simulink model "FOC_PMSM_FVSensorNew"  (R2019b)
settings: Solver=ode45  StartTime=0  StopTime=1  FixedStep=1/fs/4  MaxStep=1/fs/2  RelTol=1e-7  EnableMultiTasking=on
InitFcn:
  | Motor_parameters_Lsrpm7fw
values from neighbouring files (symbols this model uses):
  c2 = -L2/(L1^2-L2^2)    (= 10.9375)    [Motor_parameters_Lsrpm7fw.m]
  fs = 20e3    (= 20000)    [Motor_parameters_Lsrpm7fw.m]
  Iphmax = I_rated*sqrt(2)*3    [Motor_parameters_Lsrpm7fw.m]
  J = 1*1e-3    (= 0.001)    [Motor_parameters_Lsrpm7fw.m]
  Ki1 = 2    [Motor_parameters_Lsrpm7fw.m]
  Ki2 = 3000    [Motor_parameters_Lsrpm7fw.m]
  Ki_pll = Bw^2*(1.1-0.334*zeta)^2*1/(2*k1)    (= 1705731.55439)    [Motor_parameters_Lsrpm7fw.m]
  Kp1 = 0.005    [Motor_parameters_Lsrpm7fw.m]
  Kp2 = 2    [Motor_parameters_Lsrpm7fw.m]
  Kp_pll = Bw*(2.2*zeta-0.668*zeta^2)*1/(2*k1)    (= 27920.01984)    [Motor_parameters_Lsrpm7fw.m]
  Ld = 10e-3    (= 0.01)    [Motor_parameters_Lsrpm7fw.m]
  Lndd_ini = Lndmpm    (= 0.412)    [Motor_parameters_Lsrpm7fw.m]
  Lndmpm = 0.412    [Motor_parameters_Lsrpm7fw.m]
  Lq = 12.8e-3    (= 0.0128)    [Motor_parameters_Lsrpm7fw.m]
  Npp = 8/2    (= 4)    [Motor_parameters_Lsrpm7fw.m]
  Omegae_ini = 0    [Motor_parameters_Lsrpm7fw.m]
  Rs = 0.78    [Motor_parameters_Lsrpm7fw.m]
  Tl_const = Trat/nrat^2    (= 3.26530612245e-06)    [Motor_parameters_Lsrpm7fw.m]
  Trat = 10    [Motor_parameters_Lsrpm7fw.m]
  Vm = 70    [Motor_parameters_Lsrpm7fw.m]
  Vph = Vs*sqrt(2)    [Motor_parameters_Lsrpm7fw.m]
  wo = 15    [Motor_parameters_Lsrpm7fw.m]
undefined symbols (not defined in the file or in its folder): DiscIntNeverNeededParam, plecs, sigbuilder_block
libraries: simulink x1
(part 1 of 2)
settings Model: Creator=klu  LastModifiedBy=Kristina
settings SolverCC: AlgebraicLoopSolver=LineSearch
settings DataIOCC: LimitDataPoints=on  SaveFormat=Array  SignalLoggingSaveFormat=ModelDataLogs  ReturnWorkspaceOutputs=off
settings OptimizationCC: BooleanDataType=off  ExpressionDepthLimit=2147483647  InitFltsAndDblsToZero=on  LifeSpan=inf
settings DebuggingCC: AlgebraicLoopMsg=none  SaveWithParameterizedLinksMsg=none  UnderspecifiedInitializationDetection=Classic  MergeDetectMultiDrivingBlocksExec=none  SignalResolutionControl=TryResolveAllWithWarning  MultiTaskDSMMsg=warning  MultiTaskCondExecSysMsg=none  FcnCallInpInsideContextMsg=warning  StateNameClashWarn=warning  SFUnexpectedBacktrackingDiag=warning  SFNoUnconditionalDefaultTransitionDiag=warning  SFExecutionAtInitializationDiag=none  ArithmeticOperatorsInVariantConditions=warning
settings HardwareCC: ProdBitPerPointer=32  ProdBitPerSizeT=32  ProdBitPerPtrDiffT=32  ProdLargestAtomicFloat=None  ProdIntDivRoundTo=Undefined  ProdEndianess=Unspecified  ProdWordSize=32  ProdHWDeviceType=32-bit Generic
settings ModelReferenceCC: PropagateSignalLabelsOutOfModel=off
settings SFSimCC: SimUseLocalCustomCode=off  CustomCodeUndefinedFunction=UseInterfaceOnly
settings RTWCC: RTWUseLocalCustomCode=off
settings CodeAppCC: StateflowObjectComments=on
settings GRTTargetCC: TargetFcnLib=ansi_tfl_tmw.mat  TargetLangStandard=C89/C90 (ANSI)  GeneratePreprocessorConditionals=Disable all  CombineOutputUpdateFcns=off  GRTInterface=on
settings ConfigComp: CovMetricSettings=dw  CovHtmlReporting=on  CovSaveCumulativeToWorkspaceVar=on  CovSaveSingleToWorkspaceVar=on  CovExternalEMLEnable=off  CovSFcnEnable=off

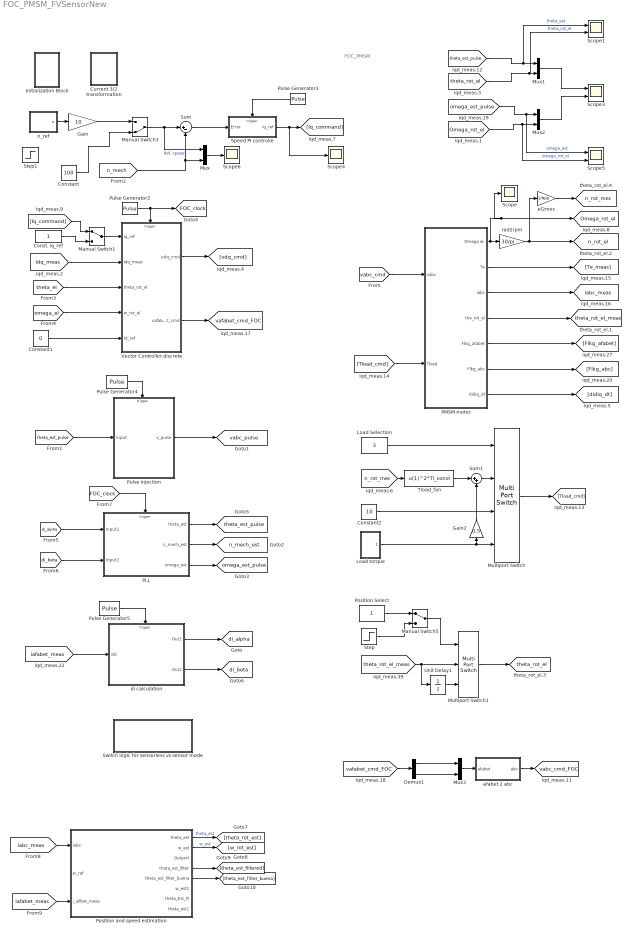
== system FOC_PMSM_FVSensorNew ==
  note: FOC_PMSM
  Const. iq_ref : Constant
  Constant : Constant  Value=100
  Constant1 : Constant  Value=0
  Constant2 : Constant  Value=10
  Current 3/2 transformation : Subsystem
      mask Display:
      | plot([0.1000    0.1357    0.1714    0.2071    0.2429    0.2786    0.3143    0.3500    0.3857    0.4214 0.4571    0.4929    0.5286    0.5643    0.6000]-0.05,0.4+0.6*[0.5000    0.5868    0.6564    0.6950    0.6950    0.6564    0.5868    0.5000    0.4132    0.3436 0.3050    0.3050    0.3436    0.4132    0.5000])
      | 
      | plot([0.1,0.9],[0.1,0.9])
      | 
      | plot([0.5,0.9],0.3*[1 1])
  Demux1 : Demux  Outputs=2
  Gain : Gain  Gain=10
  Gain2 : Gain  Gain=0.5
  Initialization Block : Subsystem  mask{init_in=Motor_parameters_Lsrpm7fw}
      mask prompts: init_in "Enter Initialization Script:"
      mask init:
      | aaa =3;
      mask Callback init_in:
      | init_script=get_param(gcb,'MaskValueString');
      | %eval(init_script);
      | %set_param(gcs,'PreLoadFcn',init_script)
      | set_param(gcs,'InitFcn',init_script)
      | 
      | % Change the parameters here;
      | Ld               = Ld;
      | Lq               = Ld;
  Load Selection : Constant  Value=3
  Load torque : Subsystem
  Manual Switch1 : ManualSwitch
  Manual Switch3 : ManualSwitch  CurrentSetting=0
  Manual Switch5 : ManualSwitch
  Multiport Switch : MultiPortSwitch
  Multiport Switch1 : MultiPortSwitch  Inputs=2
  Mux{,1..3} (4 alike) : Mux  Inputs=2
  PLL : Subsystem  TreatAsAtomicUnit=on
  PMSM motor : Subsystem
  Position Select : Constant
  Position and speed estimation : Subsystem  TreatAsAtomicUnit=on
  Pulse Generator2 : DiscretePulseGenerator  PulseType=Time based  Period=1/fs  PulseWidth=50
  Pulse Generator3 : DiscretePulseGenerator  PulseType=Time based  Period=1/fs  PulseWidth=50
  Pulse Generator4 : DiscretePulseGenerator  PulseType=Time based  Period=1/fs  PulseWidth=50  PhaseDelay=(1/fs)*0.5
  Pulse Generator5 : DiscretePulseGenerator  PulseType=Time based  Period=1/(fs*2)  PulseWidth=50
  Pulse injection : Subsystem  TreatAsAtomicUnit=on
  Scope : Scope
  Scope1 : Scope  NumInputPorts=2
  Scope3 : Scope  NumInputPorts=2
  Scope4 : Scope
  Scope5 : Scope  NumInputPorts=2
  Scope6 : Scope
  Speed PI controlle : Subsystem
  Step : Step  Time=0  Before=1  After=2  SampleTime=0
  Step1 : Step  Time=0.2  Before=100  After=100  SampleTime=0
  Sum : Sum  Inputs=|+-
  Sum1 : Sum  Inputs=|++
  Switch logic for sensorless vs sensor mode : Subsystem
  Tload_fan : Fcn  Expr=u(1)^2*Tl_const
  Unit Delay1 : UnitDelay  SampleTime=(1/fs)*4  HasFrameUpgradeWarning=on
  Vector Controller.discrete : Subsystem
  afabet 2 abc : Subsystem
  di calculation : Subsystem  TreatAsAtomicUnit=on
  el2mec : Gain  Gain=1/Npp
  n_ref : Subsystem  Tag=STV Subsys  LoadFcn=sigbuilder_block('load');  StartFcn=sigbuilder_block('start');  StopFcn=sigbuilder_block('stop');  ClipboardFcn=sigbuilder_block('clipboard');  mask(Sigbuilder block){tuvar=[0:10]}
      mask help: Sigbuilder GUI
      mask init:
      | if ~strcmp(get_param(bdroot(gcbh),'SimulationStatus'),'stopped') tuvar = sigbuilder_block('maskInit'); end
      settings: CopyFcn=sigbuilder_block('copy');  DeleteFcn=sigbuilder_block('delete');  ModelCloseFcn=sigbuilder_block('modelClose');  PreSaveFcn=sigbuilder_block('preSave');  PauseFcn=sigbuilder_block('pause')  ContinueFcn=sigbuilder_block('continue')  NameChangeFcn=sigbuilder_block('namechange');  OpenFcn=sigbuilder_block('open',[72.75 116.25 550.5 363.75 ]);  CloseFcn=sigbuilder_block('close');
      mask Display: plot(0, 0, 100, 100,[2, 2, 32, 32, 2], [68, 8, 8, 68, 68],[32, 2], [38, 38], [32, 19, 2],[53, 60, 44], [32, 17, 17, 2],[16, 16, 31, 31]);txt = getActiveGroup(gcbh);text(2, 100, txt,'verticalAlignment', 'top');
  rad2rpm : Gain  Gain=30/pi
  tag scope: FOC_clock=global, Omega_rot_el=global, di_alpha=global, di_beta=global, iabc_meas=global, n_mech_est=global, n_rot_el=global, n_rot_mec=global, omega_est_pulse=global, theta_est_pulse=global, theta_rot_el=global, theta_rot_el_meas=global, vabc_cmd_FOC=global, vabc_pulse=global, vafabet_cmd_FOC=global
  wires:
  Manual Switch1/1 -> Vector Controller.discrete/1(iq_ref)
  Const. iq_ref/1 -> Manual Switch1/2
  Sum/1 -> Speed PI controlle/1(Error)
  [idq_meas] -> Vector Controller.discrete/2(idq_meas)
  Vector Controller.discrete/1(udq_cmd) -> [vdq_cmd]
  Vector Controller.discrete/2(uafabet_cmd) -> [vafabet_cmd_FOC]
  Constant2/1 -> Multiport Switch/3
  Load torque/1(T_load) -> Multiport Switch/4, Gain2/1
  Multiport Switch/1 -> [Tload_cmd]
  [n_rot_mec] -> Tload_fan/1
  Load Selection/1 -> Multiport Switch/1
  [theta_rot_el_meas] -> Unit Delay1/1, Multiport Switch1/2
  Multiport Switch1/1 -> [theta_rot_el]
  Position Select/1 -> Manual Switch5/1
  Step/1 -> Manual Switch5/2
  Manual Switch5/1 -> Multiport Switch1/1
  n_ref/1(n) -> Gain/1
  Gain/1 -> Manual Switch3/1
  Sum1/1 -> Multiport Switch/2
  Tload_fan/1 -> Sum1/1
  [theta_el] -> Vector Controller.discrete/3(theta_rot_el)
  Constant1/1 -> Vector Controller.discrete/5(Id_ref)
  Gain2/1 -> Sum1/2
  Unit Delay1/1 -> Multiport Switch1/3
  [omega_el] -> Vector Controller.discrete/4(w_rot_el)
  PMSM motor/2(Te) -> [Te_meas]
  PMSM motor/1(Omega el.) -> Scope/1, [Omega_rot_el], rad2rpm/1
  rad2rpm/1 -> [n_rot_el], el2mec/1
  PMSM motor/5(Flkg_afabet) -> [Flkg_afabet]
  PMSM motor/6(Flkg_abc) -> [Flkg_abc]
  [Tload_cmd] -> PMSM motor/2(Tload)
  PMSM motor/3(iabc) -> [iabc_meas]
  PMSM motor/7(didiq_dt) -> [didiq_dt]
  Demux1/2 -> Mux3/2
  Demux1/1 -> Mux3/1
  [vafabet_cmd_FOC] -> Demux1/1
  afabet 2 abc/1(abc) -> [vabc_cmd_FOC]
  Mux3/1 -> afabet 2 abc/1(afabet)
  Speed PI controlle/1(iq_ref) -> Scope4/1, [Iq_command]
  [Iq_command] -> Manual Switch1/1
  el2mec/1 -> [n_rot_mec]
  Pulse Generator3/1 -> Speed PI controlle/Trigger
  Pulse Generator4/1 -> Pulse injection/Trigger
  Pulse Generator2/1 -> [FOC_clock], Vector Controller.discrete/Trigger
  [iafabet_meas] -> di calculation/1(iab)
  Pulse injection/1(v_pulse) -> [vabc_pulse]
  Manual Switch3/1 -> Mux/1, Sum/1  "Ref. speed"
  Mux/1 -> Scope6/1
  [n_mech] -> Mux/2, Sum/2
  [vabc_cmd] -> PMSM motor/1(vabc)
  Pulse Generator5/1 -> di calculation/Trigger
  PMSM motor/4(the_rot_el) -> [theta_rot_el_meas]
  PLL/1(theta_est) -> [theta_est_pulse]
  PLL/2(n_mech_est) -> [n_mech_est]
  PLL/3(omega_est) -> [omega_est_pulse]
  [theta_est_pulse] -> Pulse injection/1(Input)
  di calculation/1(Out1) -> [di_alpha]
  di calculation/2(Out2) -> [di_beta]
  [di_alpha] -> PLL/1(Input1)
  [di_beta] -> PLL/2(Input2)
  [FOC_clock] -> PLL/Trigger
  [theta_est_pulse] -> Scope1/1, Mux1/1  "theta_est"
  [theta_rot_el] -> Scope1/2, Mux1/2  "theta_rot_el"
  [omega_est_pulse] -> Scope5/1, Mux2/1  "omega_est"
  [Omega_rot_el] -> Scope5/2, Mux2/2  "omega_rot_el"
  Mux1/1 -> Scope3/1
  Mux2/1 -> Scope3/2
  Constant/1 -> Manual Switch3/2
  Position and speed estimation/2(w_est) -> [w_rot_est]  "w_est"
  Position and speed estimation/1(theta_est) -> [theta_rot_est]  "theta_est"
  Position and speed estimation/4(theta_est_filter) -> [theta_est_filtered]
  [iabc_meas] -> Position and speed estimation/1(Iabc)
  Position and speed estimation/5(theta_est_filter_buena) -> [theta_est_filter_buena]
  [iafabet_meas] -> Position and speed estimation/3(i_alfbet_meas)

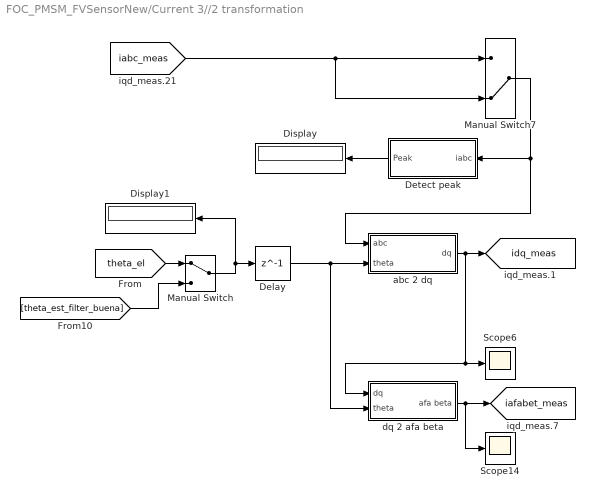
== system FOC_PMSM_FVSensorNew/Current 3//2 transformation ==
  Delay : Delay  DelayLength=1
  Detect peak : Subsystem
  Display : Display
  Display1 : Display
  Manual Switch : ManualSwitch
  Manual Switch7 : ManualSwitch  CurrentSetting=0
  Scope14 : Scope
  Scope6 : Scope
  abc 2 dq : Subsystem
  dq 2 afa beta : Subsystem
  tag scope: iafabet_meas=global, idq_meas=global
  wires:
  abc 2 dq/1(dq) -> [idq_meas], Scope6/1, dq 2 afa beta/1(dq)
  dq 2 afa beta/1(afa beta) -> [iafabet_meas], Scope14/1
  Manual Switch7/1 -> abc 2 dq/1(abc), Detect peak/1(iabc)
  Detect peak/1(Peak) -> Display/1
  [iabc_meas] -> Manual Switch7/1, Manual Switch7/2
  Delay/1 -> abc 2 dq/2(theta), dq 2 afa beta/2(theta)
  [theta_el] -> Manual Switch/1
  Manual Switch/1 -> Display1/1, Delay/1
  [theta_est_filter_buena] -> Manual Switch/2

== system FOC_PMSM_FVSensorNew/Initialization Block ==

== system FOC_PMSM_FVSensorNew/Load torque ==
  Add : Sum  Inputs=+++
  Scope2 : Scope
  Step Load torque 1 : Step  Time=2  After=Trat  SampleTime=0
  Step Load torque2 : Step  Time=4  After=-Trat/2  SampleTime=0
  Tload : Constant  Value=0
  T_load : Outport  VectorParamsAs1DForOutWhenUnconnected=off
  wires:
  Tload/1 -> Add/1
  Step Load torque 1/1 -> Add/2
  Step Load torque2/1 -> Add/3
  Add/1 -> T_load/1, Scope2/1

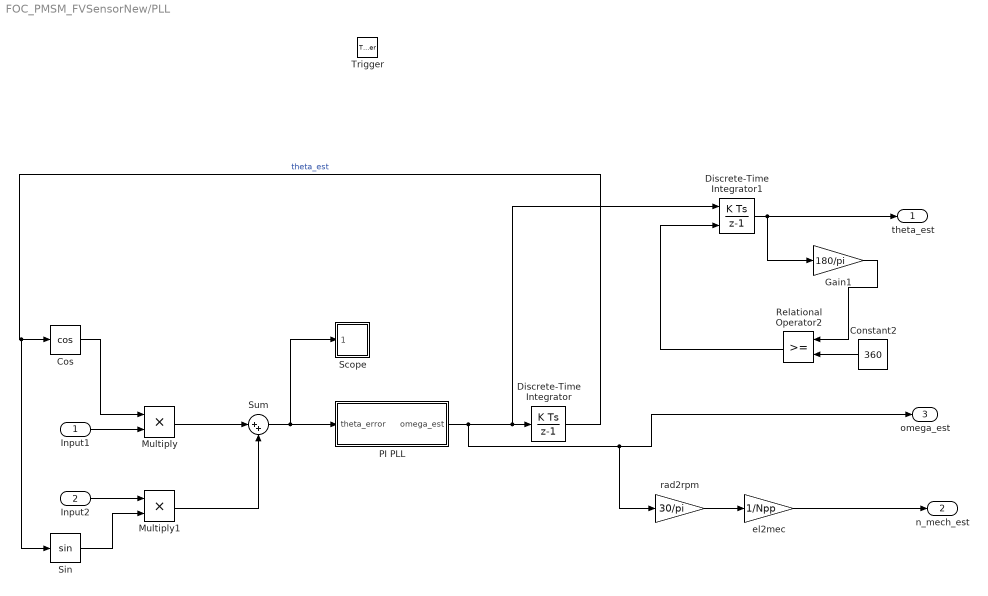
== system FOC_PMSM_FVSensorNew/PLL ==
  Input1 : Inport
  Input2 : Inport  Port=2
  Trigger : TriggerPort  VariantControl=Variant
  Constant2 : Constant  Value=360
  Cos : Trigonometry  Operator=cos
  Discrete-Time Integrator : DiscreteIntegrator  SampleTime=-1  ICPrevOutput=DiscIntNeverNeededParam  ICPrevScaledInput=DiscIntNeverNeededParam
  Discrete-Time Integrator1 : DiscreteIntegrator  ExternalReset=rising  SampleTime=-1  ICPrevOutput=DiscIntNeverNeededParam  ICPrevScaledInput=DiscIntNeverNeededParam
  Gain1 : Gain  Gain=180/pi
  Multiply : Product
  Multiply1 : Product
  PI PLL : Subsystem
  Relational Operator2 : RelationalOperator  OutDataTypeStr=boolean  RndMeth=Nearest
  Scope : Subsystem  LoadFcn=plecs('sl', 300);  InitFcn=plecs('sl', 314);  StartFcn=plecs('sl', 308);  StopFcn=plecs('sl', 309);  mask{Settings=<binary blob, 232 chars, not shown>}
      mask init:
      | plecs('sl', 315);
      settings: CopyFcn=plecs('sl', 303);  DeleteFcn=plecs('sl', 305);  UndoDeleteFcn=plecs('sl', 306);  PreSaveFcn=plecs('sl', 311);  NameChangeFcn=plecs('sl', 310);  DestroyFcn=plecs('sl', 307);  OpenFcn=plecs('sl', 302);  ErrorFcn=plerrorfcn
      mask Display: plot([0.1 0.9 0.9 0.1 0.1], [0.9 0.9 0.5 0.5 0.9])
  Sin : Trigonometry
  Sum : Sum  Inputs=|++
  el2mec : Gain  Gain=1/Npp
  rad2rpm : Gain  Gain=30/pi
  theta_est : Outport  VectorParamsAs1DForOutWhenUnconnected=off
  n_mech_est : Outport  Port=2  VectorParamsAs1DForOutWhenUnconnected=off
  omega_est : Outport  Port=3  VectorParamsAs1DForOutWhenUnconnected=off
  wires:
  el2mec/1 -> n_mech_est/1
  Sum/1 -> Scope/1(1), PI PLL/1(theta_error)
  Multiply/1 -> Sum/1
  Relational Operator2/1 -> Discrete-Time Integrator1/2
  Input2/1 -> Multiply1/1
  Gain1/1 -> Relational Operator2/1
  Discrete-Time Integrator1/1 -> Gain1/1, theta_est/1
  Cos/1 -> Multiply/1
  Sin/1 -> Multiply1/2
  Input1/1 -> Multiply/2
  rad2rpm/1 -> el2mec/1
  Discrete-Time Integrator/1 -> Sin/1, Cos/1  "theta_est"
  PI PLL/1(omega_est) -> rad2rpm/1, omega_est/1, Discrete-Time Integrator1/1, Discrete-Time Integrator/1
  Constant2/1 -> Relational Operator2/2
  Multiply1/1 -> Sum/2

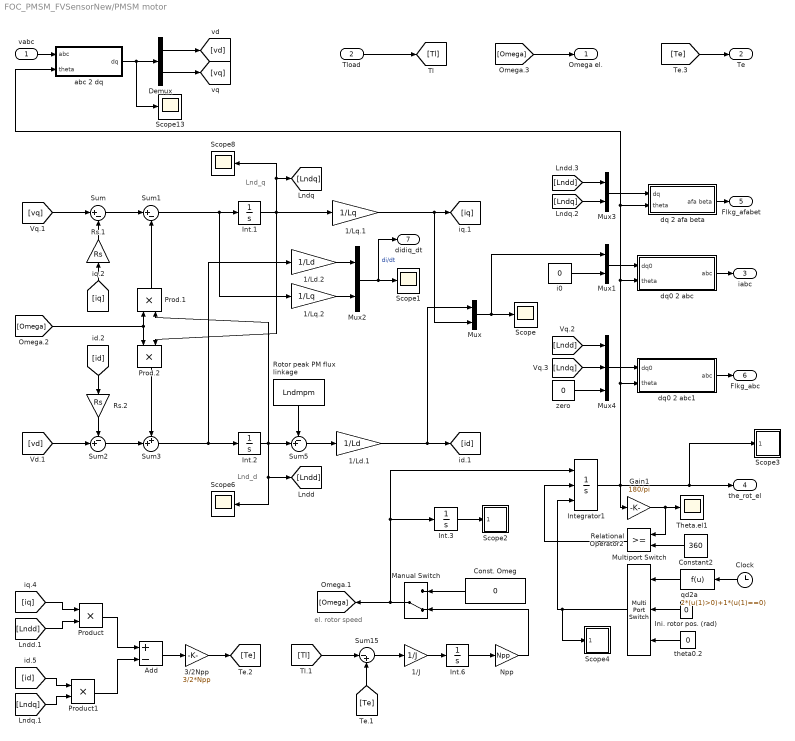
== system FOC_PMSM_FVSensorNew/PMSM motor ==
  note: Lnd_d
  note: Lnd_q
  note: el. rotor speed
  vabc : Inport
  Tload : Inport  Port=2
  1/J : Gain  Gain=1/J
  1/Ld.1 : Gain  Gain=1/Ld
  1/Ld.2 : Gain  Gain=1/Ld
  1/Lq.1 : Gain  Gain=1/Lq
  1/Lq.2 : Gain  Gain=1/Lq
  3/2Npp : Gain  Gain=3/2*Npp
  Add : Sum  Inputs=+-
  Clock : Clock
  Const. Omeg : Constant  Value=0
  Constant2 : Constant  Value=360
  Demux : Demux  Outputs=2
  Gain1 : Gain  Gain=180/pi
  Ini. rotor pos. (rad) : Constant  Value=0
  Int.1 : Integrator
  Int.2 : Integrator  InitialCondition=Lndd_ini
  Int.3 : Integrator  InitialCondition=Omegae_ini/Npp
  Int.6 : Integrator  InitialCondition=Omegae_ini/Npp
  Integrator1 : Integrator  ExternalReset=rising  InitialConditionSource=external  InitialCondition=pi/3
  Manual Switch : ManualSwitch  CurrentSetting=0
  Multiport Switch : MultiPortSwitch  Inputs=2
  Mux{,1..3} (4 alike) : Mux  Inputs=2
  Mux4 : Mux  Inputs=3
  Npp : Gain  Gain=Npp
  Prod.1 : Product  RndMeth=Zero
  Prod.2 : Product  RndMeth=Zero
  Product : Product  RndMeth=Zero
  Product1 : Product  RndMeth=Zero
  Relational Operator2 : RelationalOperator  OutDataTypeStr=boolean  RndMeth=Nearest
  Rotor peak PM flux linkage : Constant  Value=Lndmpm
  Rs.1 : Gain  Gain=Rs
  Rs.2 : Gain  Gain=Rs
  Scope{,1,6,8,13} (5 alike) : Scope
  Scope2 : Subsystem  LoadFcn=plecs('sl', 300);  InitFcn=plecs('sl', 314);  StartFcn=plecs('sl', 308);  StopFcn=plecs('sl', 309);  mask{Settings=<binary blob, 1052 chars, not shown>}
      mask init:
      | plecs('sl', 315);
      settings: CopyFcn=plecs('sl', 303);  DeleteFcn=plecs('sl', 305);  UndoDeleteFcn=plecs('sl', 306);  PreSaveFcn=plecs('sl', 311);  NameChangeFcn=plecs('sl', 310);  DestroyFcn=plecs('sl', 307);  OpenFcn=plecs('sl', 302);  ErrorFcn=plerrorfcn
      mask Display: plot([0.1 0.9 0.9 0.1 0.1], [0.9 0.9 0.5 0.5 0.9])
  Scope3 : Subsystem  LoadFcn=plecs('sl', 300);  InitFcn=plecs('sl', 314);  StartFcn=plecs('sl', 308);  StopFcn=plecs('sl', 309);  mask{Settings=<binary blob, 1052 chars, not shown>}
      mask init:
      | plecs('sl', 315);
      settings: CopyFcn=plecs('sl', 303);  DeleteFcn=plecs('sl', 305);  UndoDeleteFcn=plecs('sl', 306);  PreSaveFcn=plecs('sl', 311);  NameChangeFcn=plecs('sl', 310);  DestroyFcn=plecs('sl', 307);  OpenFcn=plecs('sl', 302);  ErrorFcn=plerrorfcn
      mask Display: plot([0.1 0.9 0.9 0.1 0.1], [0.9 0.9 0.5 0.5 0.9])
  Scope4 : Subsystem  LoadFcn=plecs('sl', 300);  InitFcn=plecs('sl', 314);  StartFcn=plecs('sl', 308);  StopFcn=plecs('sl', 309);  mask{Settings=<binary blob, 1052 chars, not shown>}
      mask init:
      | plecs('sl', 315);
      settings: CopyFcn=plecs('sl', 303);  DeleteFcn=plecs('sl', 305);  UndoDeleteFcn=plecs('sl', 306);  PreSaveFcn=plecs('sl', 311);  NameChangeFcn=plecs('sl', 310);  DestroyFcn=plecs('sl', 307);  OpenFcn=plecs('sl', 302);  ErrorFcn=plerrorfcn
      mask Display: plot([0.1 0.9 0.9 0.1 0.1], [0.9 0.9 0.5 0.5 0.9])
  Sum : Sum  Inputs=|+-
  Sum1 : Sum  Inputs=|+-
  Sum15 : Sum  Inputs=|-+
  Sum2 : Sum  Inputs=-+|
  Sum3 : Sum  Inputs=++|
  Sum5 : Sum  Inputs=-+|
  Theta.el1 : Scope
  abc 2 dq : Subsystem
  dq 2 afa beta : Subsystem
  dq0 2 abc : Subsystem
  dq0 2 abc1 : Subsystem
  i0 : Constant  Value=0
  qd2a : Fcn  Expr=2*(u(1)>0)+1*(u(1)==0)
  theta0.2 : Constant  Value=0
  zero : Constant  Value=0
  Omega el. : Outport  VectorParamsAs1DForOutWhenUnconnected=off
  Te : Outport  Port=2  VectorParamsAs1DForOutWhenUnconnected=off
  iabc : Outport  Port=3  VectorParamsAs1DForOutWhenUnconnected=off
  the_rot_el : Outport  Port=4  VectorParamsAs1DForOutWhenUnconnected=off
  Flkg_afabet : Outport  Port=5  VectorParamsAs1DForOutWhenUnconnected=off
  Flkg_abc : Outport  Port=6  VectorParamsAs1DForOutWhenUnconnected=off
  didiq_dt : Outport  Port=7  VectorParamsAs1DForOutWhenUnconnected=off
  wires:
  3/2Npp/1 -> [Te]
  Add/1 -> 3/2Npp/1
  Sum5/1 -> 1/Ld.1/1
  Rotor peak PM flux linkage/1 -> Sum5/1
  [Omega] -> Omega el./1
  [Te] -> Te/1
  Product1/1 -> Add/2
  Product/1 -> Add/1
  [Lndq] -> Product1/2
  [id] -> Product1/1
  [Te] -> Sum15/2
  Int.6/1 -> Npp/1
  1/J/1 -> Int.6/1
  Sum15/1 -> 1/J/1
  [Tl] -> Sum15/1
  Mux/1 -> Scope/1, Mux1/1
  [Omega] -> Prod.2/1, Prod.1/1
  Sum3/1 -> Int.2/1, 1/Ld.2/1
  Prod.2/1 -> Sum3/1
  Sum2/1 -> Sum3/2
  [id] -> Rs.2/1
  Rs.2/1 -> Sum2/1
  [vd] -> Sum2/2
  1/Ld.1/1 -> [id], Mux/1
  Int.2/1 -> [Lndd], Scope6/1, Sum5/2, Prod.1/2
  [iq] -> Rs.1/1
  1/Lq.1/1 -> [iq], Mux/2
  Prod.1/1 -> Sum1/2
  Sum1/1 -> Int.1/1, 1/Lq.2/1
  Int.1/1 -> 1/Lq.1/1, Prod.2/2, Scope8/1, [Lndq]
  Sum/1 -> Sum1/1
  Rs.1/1 -> Sum/2
  [vq] -> Sum/1
  Tload/1 -> [Tl]
  Demux/2 -> [vq]
  Demux/1 -> [vd]
  i0/1 -> Mux1/2
  Mux1/1 -> dq0 2 abc/1(dq0)
  dq0 2 abc/1(abc) -> iabc/1
  vabc/1 -> abc 2 dq/1(abc)
  abc 2 dq/1(dq) -> Demux/1, Scope13/1
  Integrator1/1 -> Scope3/1(1), the_rot_el/1, dq0 2 abc/2(theta), dq 2 afa beta/2(theta), abc 2 dq/2(theta), dq0 2 abc1/2(theta), Gain1/1
  1/Ld.2/1 -> Mux2/1
  1/Lq.2/1 -> Mux2/2
  Mux2/1 -> didiq_dt/1, Scope1/1  "di/dt"
  Mux3/1 -> dq 2 afa beta/1(dq)
  [Lndd] -> Mux3/1
  [Lndq] -> Mux3/2
  dq 2 afa beta/1(afa beta) -> Flkg_afabet/1
  [Lndd] -> Mux4/1
  [Lndq] -> Mux4/2
  Mux4/1 -> dq0 2 abc1/1(dq0)
  dq0 2 abc1/1(abc) -> Flkg_abc/1
  zero/1 -> Mux4/3
  Gain1/1 -> Theta.el1/1, Relational Operator2/1
  Constant2/1 -> Relational Operator2/2
  [iq] -> Product/1
  [Lndd] -> Product/2
  Relational Operator2/1 -> Integrator1/2
  Ini. rotor pos. (rad)/1 -> Multiport Switch/2
  theta0.2/1 -> Multiport Switch/3
  qd2a/1 -> Multiport Switch/1
  Clock/1 -> qd2a/1
  Multiport Switch/1 -> Scope4/1(1), Integrator1/3
  Const. Omeg/1 -> Manual Switch/1
  Npp/1 -> Manual Switch/2
  Manual Switch/1 -> Int.3/1, Integrator1/1, [Omega]
  Int.3/1 -> Scope2/1(1)

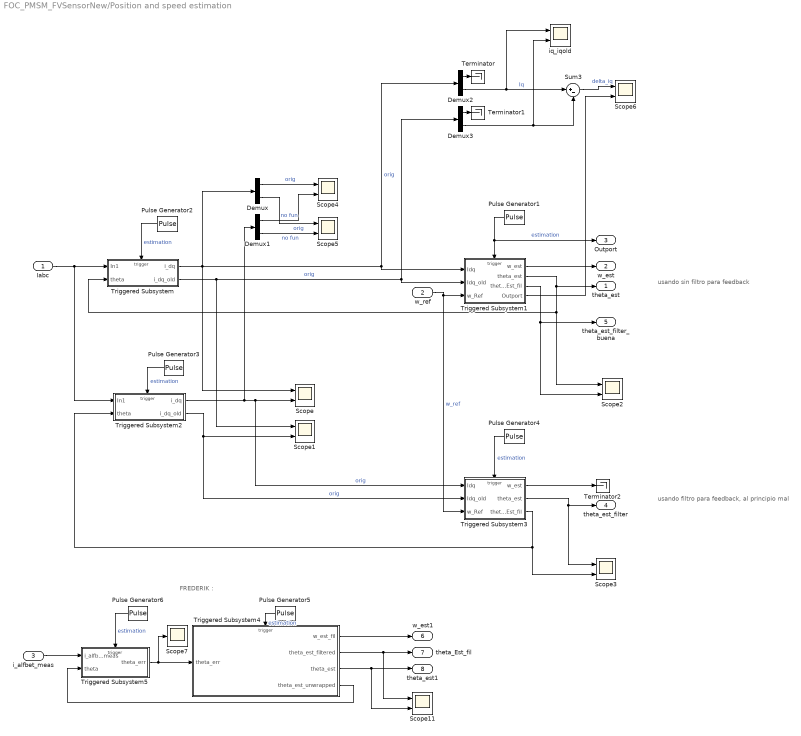
== system FOC_PMSM_FVSensorNew/Position and speed estimation ==
  note: FREDERIK :
  note: usando filtro para feedback, al principio mal
  note: usando sin filtro para feedback
  Iabc : Inport
  w_ref : Inport  Port=2
  i_alfbet_meas : Inport  Port=3
  Demux{,1..3} (4 alike) : Demux  Outputs=2
  Pulse Generator1 : DiscretePulseGenerator  PulseType=Time based  Period=2/fs  PulseWidth=50  PhaseDelay=1/fs
  Pulse Generator2 : DiscretePulseGenerator  PulseType=Time based  Period=1/fs  PulseWidth=50
  Pulse Generator3 : DiscretePulseGenerator  PulseType=Time based  Period=1/fs  PulseWidth=50
  Pulse Generator4 : DiscretePulseGenerator  PulseType=Time based  Period=2/fs  PulseWidth=50  PhaseDelay=1/fs
  Pulse Generator5 : DiscretePulseGenerator  PulseType=Time based  Period=2/fs  PulseWidth=50  PhaseDelay=1/fs
  Pulse Generator6 : DiscretePulseGenerator  PulseType=Time based  Period=1/fs  PulseWidth=50
  Scope{,1..6,11} (8 alike) : Scope  NumInputPorts=2
  Scope7 : Scope
  Sum3 : Sum  Inputs=|+-
  Terminator : Terminator
  Terminator1 : Terminator
  Terminator2 : Terminator
  Triggered Subsystem : Subsystem  TreatAsAtomicUnit=on
  Triggered Subsystem1 : Subsystem  TreatAsAtomicUnit=on
  Triggered Subsystem2 : Subsystem  TreatAsAtomicUnit=on
  Triggered Subsystem3 : Subsystem  TreatAsAtomicUnit=on
  Triggered Subsystem4 : Subsystem  TreatAsAtomicUnit=on
  Triggered Subsystem5 : Subsystem  TreatAsAtomicUnit=on
  iq_iqold : Scope  NumInputPorts=2
  theta_est : Outport
  w_est : Outport  Port=2
  Outport : Outport  Port=3
  theta_est_filter : Outport  Port=4
  theta_est_filter_buena : Outport  Port=5
  w_est1 : Outport  Port=6
  theta_Est_fil : Outport  Port=7
  theta_est1 : Outport  Port=8
  wires:
  Pulse Generator1/1 -> Triggered Subsystem1/Trigger, Outport/1  "estimation"
  Triggered Subsystem1/1(w_est) -> w_est/1
  Triggered Subsystem/2(i_dq_old) -> Scope1/1, Demux3/1, Triggered Subsystem1/2(Idq_old)  "orig"
  Triggered Subsystem1/2(theta_est) -> Scope2/1, Triggered Subsystem/2(theta), theta_est/1
  Triggered Subsystem/1(i_dq) -> Scope/1, Demux/1, Demux2/1, Triggered Subsystem1/1(Idq)  "orig"
  w_ref/1 -> Triggered Subsystem3/3(w_Ref), Triggered Subsystem1/3(w_Ref)  "w_ref"
  Pulse Generator2/1 -> Triggered Subsystem/Trigger  "estimation"
  Triggered Subsystem1/3(theta_Est_fil) -> theta_est_filter_buena/1, Scope2/2
  Pulse Generator3/1 -> Triggered Subsystem2/Trigger  "estimation"
  Demux/1 -> Scope4/1  "orig"
  Demux1/1 -> Scope4/2  "no fun"
  Demux/2 -> Scope5/1  "orig"
  Demux1/2 -> Scope5/2  "no fun"
  Pulse Generator4/1 -> Triggered Subsystem3/Trigger  "estimation"
  Triggered Subsystem3/3(theta_Est_fil) -> Triggered Subsystem2/2(theta), Scope3/2
  Triggered Subsystem2/2(i_dq_old) -> Triggered Subsystem3/2(Idq_old), Scope1/2  "orig"
  Triggered Subsystem2/1(i_dq) -> Triggered Subsystem3/1(Idq), Scope/2, Demux1/1  "orig"
  Triggered Subsystem3/2(theta_est) -> Scope3/1, theta_est_filter/1
  Triggered Subsystem3/1(w_est) -> Terminator2/1
  Demux2/1 -> Terminator/1
  Demux3/1 -> Terminator1/1
  Demux2/2 -> iq_iqold/1, Sum3/1  "Iq"
  Demux3/2 -> iq_iqold/2, Sum3/2
  Sum3/1 -> Scope6/1  "delta_iq"
  Triggered Subsystem1/4(Outport) -> Scope6/2
  Iabc/1 -> Triggered Subsystem2/1(In1), Triggered Subsystem/1(In1)
  Triggered Subsystem4/3(theta_est) -> Scope11/2, theta_est1/1
  i_alfbet_meas/1 -> Triggered Subsystem5/1(i_alfbet_meas)
  Triggered Subsystem4/1(w_est_fil) -> w_est1/1
  Triggered Subsystem4/2(theta_est_filtered) -> Scope11/1, theta_Est_fil/1
  Pulse Generator5/1 -> Triggered Subsystem4/Trigger  "estimation"
  Pulse Generator6/1 -> Triggered Subsystem5/Trigger  "estimation"
  Triggered Subsystem5/1(theta_err) -> Scope7/1, Triggered Subsystem4/1(theta_err)
  Triggered Subsystem4/4(theta_est_unwrapped) -> Triggered Subsystem5/2(theta)

== system FOC_PMSM_FVSensorNew/Pulse injection ==
  Input : Inport
  Trigger : TriggerPort  VariantControl=Variant
  Constant : Constant  Value=0
  Constant1 : Constant  Value=Vm
  Mux : Mux  Inputs=2
  afabet 2 abc : Subsystem
  dq 2 afa beta : Subsystem
  v_pulse : Outport  VectorParamsAs1DForOutWhenUnconnected=off
  wires:
  Constant/1 -> Mux/1
  Constant1/1 -> Mux/2
  Mux/1 -> dq 2 afa beta/1(dq)
  dq 2 afa beta/1(afa beta) -> afabet 2 abc/1(afabet)
  afabet 2 abc/1(abc) -> v_pulse/1
  Input/1 -> dq 2 afa beta/2(theta)

== system FOC_PMSM_FVSensorNew/Speed PI controlle ==
  Error : Inport
  Trigger : TriggerPort  VariantControl=(inherit)
  Discrete-Time Integrator : DiscreteIntegrator  SampleTime=-1  ICPrevOutput=DiscIntNeverNeededParam  ICPrevScaledInput=DiscIntNeverNeededParam
  Kp : Gain  Gain=Kp1
  Sum1 : Sum  Inputs=|++
  ki : Gain  Gain=Ki1
  iq_ref : Outport  VectorParamsAs1DForOutWhenUnconnected=off
  wires:
  Kp/1 -> Sum1/1
  ki/1 -> Discrete-Time Integrator/1
  Discrete-Time Integrator/1 -> Sum1/2
  Sum1/1 -> iq_ref/1
  Error/1 -> Kp/1, ki/1

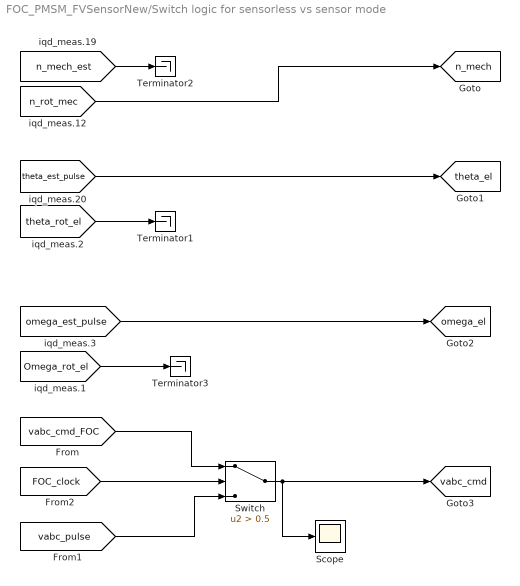
== system FOC_PMSM_FVSensorNew/Switch logic for sensorless vs sensor mode ==
  Scope : Scope
  Switch : Switch  Criteria=u2 > Threshold  Threshold=0.5
  Terminator1 : Terminator
  Terminator2 : Terminator
  Terminator3 : Terminator
  tag scope: n_mech=global, omega_el=global, theta_el=global, vabc_cmd=global
  wires:
  [n_rot_mec] -> [n_mech]
  [theta_est_pulse] -> [theta_el]
  [vabc_cmd_FOC] -> Switch/1
  [vabc_pulse] -> Switch/3
  [FOC_clock] -> Switch/2
  Switch/1 -> Scope/1, [vabc_cmd]
  [omega_est_pulse] -> [omega_el]
  [theta_rot_el] -> Terminator1/1
  [n_mech_est] -> Terminator2/1
  [Omega_rot_el] -> Terminator3/1

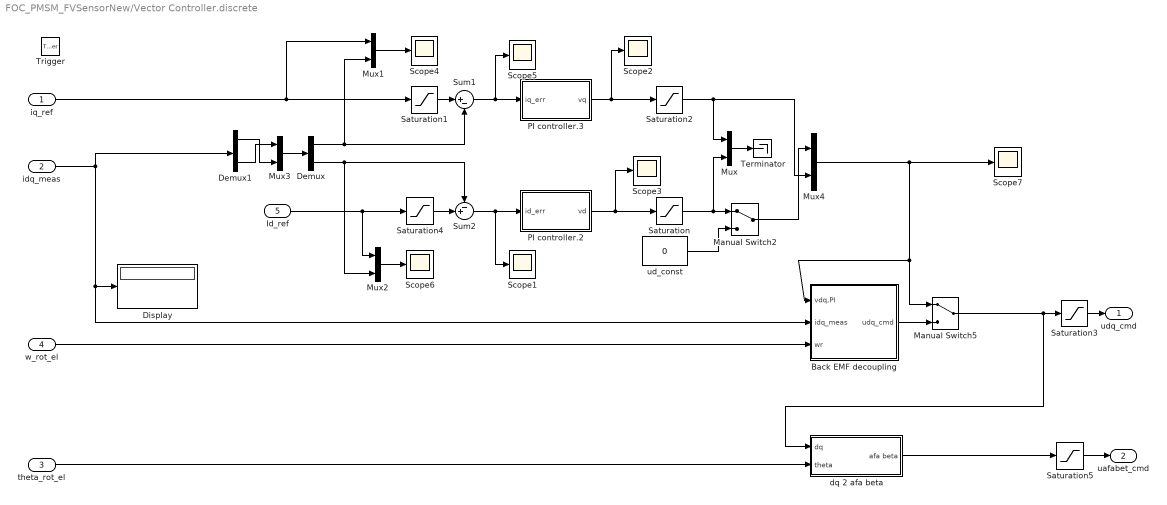
== system FOC_PMSM_FVSensorNew/Vector Controller.discrete ==
  iq_ref : Inport
  idq_meas : Inport  Port=2
  theta_rot_el : Inport  Port=3
  w_rot_el : Inport  Port=4
  Id_ref : Inport  Port=5
  Trigger : TriggerPort  VariantControl=(inherit)
  Back EMF decoupling : Subsystem
  Demux : Demux  Outputs=2
  Demux1 : Demux  Outputs=2
  Display : Display
  Manual Switch2 : ManualSwitch
  Manual Switch5 : ManualSwitch
  Mux{,1..4} (5 alike) : Mux  Inputs=2
  PI controller.2 : Subsystem
  PI controller.3 : Subsystem
  Saturation{,2..3,5} (4 alike) : Saturate  UpperLimit=Vph  LowerLimit=-Vph
  Saturation1 : Saturate  UpperLimit=Iphmax  LowerLimit=-Iphmax
  Saturation4 : Saturate  UpperLimit=Iphmax  LowerLimit=-Iphmax
  Scope{1..7} (7 alike) : Scope
  Sum1 : Sum  Inputs=|+-
  Sum2 : Sum  Inputs=-+|
  Terminator : Terminator
  dq 2 afa beta : Subsystem
  ud_const : Constant  Value=0
  udq_cmd : Outport  VectorParamsAs1DForOutWhenUnconnected=off
  uafabet_cmd : Outport  Port=2  VectorParamsAs1DForOutWhenUnconnected=off
  wires:
  Saturation4/1 -> Sum2/2
  Saturation/1 -> Mux/2, Manual Switch2/1
  Mux/1 -> Terminator/1
  PI controller.3/1(vq) -> Scope2/1, Saturation2/1
  Demux/1 -> Sum1/2, Mux1/2
  PI controller.2/1(vd) -> Saturation/1, Scope3/1
  Demux/2 -> Sum2/1, Mux2/2
  Sum1/1 -> Scope5/1, PI controller.3/1(iq_err)
  iq_ref/1 -> Mux1/1, Saturation1/1
  Sum2/1 -> Scope1/1, PI controller.2/1(id_err)
  Id_ref/1 -> Saturation4/1, Mux2/1
  Mux1/1 -> Scope4/1
  Saturation1/1 -> Sum1/1
  Mux2/1 -> Scope6/1
  Saturation2/1 -> Mux/1, Mux4/2
  Manual Switch2/1 -> Mux4/1
  ud_const/1 -> Manual Switch2/2
  Demux1/2 -> Mux3/1
  Demux1/1 -> Mux3/2
  theta_rot_el/1 -> dq 2 afa beta/2(theta)
  dq 2 afa beta/1(afa beta) -> Saturation5/1
  w_rot_el/1 -> Back EMF decoupling/3(wr)
  Back EMF decoupling/1(udq_cmd) -> Manual Switch5/2
  Mux4/1 -> Scope7/1, Manual Switch5/1, Back EMF decoupling/1(vdq,PI)
  Manual Switch5/1 -> dq 2 afa beta/1(dq), Saturation3/1
  Mux3/1 -> Demux/1
  idq_meas/1 -> Demux1/1, Display/1, Back EMF decoupling/2(idq_meas)
  Saturation3/1 -> udq_cmd/1
  Saturation5/1 -> uafabet_cmd/1

== system FOC_PMSM_FVSensorNew/afabet 2 abc ==
  afabet : Inport
  Constant : Constant  Value=0
  Mux1 : Mux  Inputs=2
  Mux2 : Mux  Inputs=3
  qd2a : Fcn  Expr=u(1)+u(3)
  qd2b : Fcn  Expr=u(1)*cos(2/3*pi)+u(2)*sin(2/3*pi)+u(3)
  qd2c : Fcn  Expr=u(1)*cos(2/3*pi)-u(2)*sin(2/3*pi)+u(3)
  abc : Outport  VectorParamsAs1DForOutWhenUnconnected=off
  wires:
  Constant/1 -> Mux1/2
  qd2c/1 -> Mux2/3
  afabet/1 -> Mux1/1
  Mux1/1 -> qd2c/1, qd2b/1, qd2a/1
  qd2a/1 -> Mux2/1
  qd2b/1 -> Mux2/2
  Mux2/1 -> abc/1

== system FOC_PMSM_FVSensorNew/di calculation ==
  iab : Inport
  Trigger : TriggerPort  VariantControl=Variant
  Delay2 : Delay  DelayLength=1
  Delay3 : Delay  DelayLength=1
  Demux : Demux  Outputs=2
  Scope : Scope  NumInputPorts=2
  Subtract : Sum  Inputs=+-
  Subtract1 : Sum  Inputs=+-
  Out1 : Outport  VectorParamsAs1DForOutWhenUnconnected=off
  Out2 : Outport  Port=2  VectorParamsAs1DForOutWhenUnconnected=off
  wires:
  Demux/1 -> Scope/1, Subtract/1, Delay2/1  "ia0"
  Demux/2 -> Delay3/1, Subtract1/1  "ib0"
  iab/1 -> Demux/1
  Delay2/1 -> Scope/2, Subtract/2  "ia1"
  Delay3/1 -> Subtract1/2  "ib1"
  Subtract/1 -> Out1/1
  Subtract1/1 -> Out2/1

== system FOC_PMSM_FVSensorNew/n_ref ==
  Demux : Demux  Tag=STV Demux  Outputs=1
  FromWs : FromWorkspace  Tag=STV FromWs  VariableName=tuvar  SampleTime=0
      SigBuilderData=|
      | common.afterFinalStr = 'Extrapolate'
      | common.sampleTime = 0
      | dataSet.timeRange = [0 10]
      | dataSet.name = 'Group 1'
      | sbobj.Groups.Name = 'Group 1'
      | sbobj.Groups.Signals.Name = 'n'
      | sbobj.Groups.Signals.XData = [0 1 1 6 6 7 10]
      | sbobj.Groups.Signals.YData = [0 0 0.995 0.995 1 0.39 0.1]
  n : Outport  Tag=STV Outport  VectorParamsAs1DForOutWhenUnconnected=off
  wires:
  Demux/1 -> n/1
  FromWs/1 -> Demux/1

== system FOC_PMSM_FVSensorNew/Current 3//2 transformation/Detect peak ==
  iabc : Inport
  Clock : Clock
  Compare To Constant : simulink/Logic and Bit Operations/Compare To Constant  relop=>=  const=2  OutDataTypeStr=uint8  ZeroCross=off
  Demux1 : Demux  Outputs=3
  MinMax : MinMax  Function=max  Inputs=2
  Product : Product  RndMeth=Zero
  Terminator : Terminator
  Terminator1 : Terminator
  Unit Delay : UnitDelay  SampleTime=1/5e3  HasFrameUpgradeWarning=on
  Peak : Outport  VectorParamsAs1DForOutWhenUnconnected=off
  wires:
  iabc/1 -> Demux1/1
  Demux1/3 -> Terminator/1
  Demux1/2 -> Terminator1/1
  Clock/1 -> Compare To Constant/1
  Compare To Constant/1 -> Product/1
  Demux1/1 -> Product/2
  MinMax/1 -> Peak/1, Unit Delay/1
  Product/1 -> MinMax/1
  Unit Delay/1 -> MinMax/2

== system FOC_PMSM_FVSensorNew/Current 3//2 transformation/abc 2 dq ==
  abc : Inport
  theta : Inport  Port=2
  Mux1 : Mux  Inputs=2
  Mux2 : Mux  Inputs=2
  abc2d : Fcn  Expr=2/3*(u(1)*cos(u(4))+u(2)*cos(u(4)-2*pi/3)+u(3)*cos(u(4)-4*pi/3))
  abc2q : Fcn  Expr=-1*2/3*(u(1)*sin(u(4))+u(2)*sin(u(4)-2*pi/3)+u(3)*sin(u(4)-4*pi/3))
  dq : Outport  VectorParamsAs1DForOutWhenUnconnected=off
  wires:
  Mux2/1 -> dq/1
  abc2q/1 -> Mux2/2
  abc2d/1 -> Mux2/1
  Mux1/1 -> abc2q/1, abc2d/1
  theta/1 -> Mux1/2
  abc/1 -> Mux1/1

== system FOC_PMSM_FVSensorNew/Current 3//2 transformation/dq 2 afa beta ==
  dq : Inport
  theta : Inport  Port=2
  Mux1 : Mux  Inputs=2
  Mux2 : Mux  Inputs=2
  dq2afa : Fcn  Expr=u(1)*cos(u(3))-u(2)*sin(u(3))
  dq2beta : Fcn  Expr=u(1)*sin(u(3))+u(2)*cos(u(3))
  afa beta : Outport  VectorParamsAs1DForOutWhenUnconnected=off
  wires:
  dq/1 -> Mux1/1
  theta/1 -> Mux1/2
  Mux1/1 -> dq2beta/1, dq2afa/1
  dq2afa/1 -> Mux2/1
  dq2beta/1 -> Mux2/2
  Mux2/1 -> afa beta/1

== system FOC_PMSM_FVSensorNew/PLL/PI PLL ==
  theta_error : Inport
  Discrete-Time Integrator : DiscreteIntegrator  SampleTime=-1  ICPrevOutput=DiscIntNeverNeededParam  ICPrevScaledInput=DiscIntNeverNeededParam
  Kp : Gain  Gain=Kp_pll
  Sum1 : Sum  Inputs=|++
  ki : Gain  Gain=Ki_pll
  omega_est : Outport  VectorParamsAs1DForOutWhenUnconnected=off
  wires:
  Sum1/1 -> omega_est/1
  Discrete-Time Integrator/1 -> Sum1/2
  ki/1 -> Discrete-Time Integrator/1
  Kp/1 -> Sum1/1
  theta_error/1 -> ki/1, Kp/1

== system FOC_PMSM_FVSensorNew/PLL/Scope ==
  1 : Inport
  " InputMux " : Subsystem
      mask Display: disp('Mux')
  " S-Function " : S-Function  FunctionName=plecs  SFunctionDeploymentMode=off  EnableBusSupport=off
  wires:
  1/1 -> " InputMux "/1(In1)
  " InputMux "/1(Out) -> " S-Function "/1

== system FOC_PMSM_FVSensorNew/PMSM motor/Scope2 ==
  1 : Inport
  " InputMux " : Subsystem
      mask Display: disp('Mux')
  " S-Function " : S-Function  FunctionName=plecs  SFunctionDeploymentMode=off  EnableBusSupport=off
  wires:
  1/1 -> " InputMux "/1(In1)
  " InputMux "/1(Out) -> " S-Function "/1

== system FOC_PMSM_FVSensorNew/PMSM motor/Scope3 ==
  1 : Inport
  " InputMux " : Subsystem
      mask Display: disp('Mux')
  " S-Function " : S-Function  FunctionName=plecs  SFunctionDeploymentMode=off  EnableBusSupport=off
  wires:
  " InputMux "/1(Out) -> " S-Function "/1
  1/1 -> " InputMux "/1(In1)

== system FOC_PMSM_FVSensorNew/PMSM motor/Scope4 ==
  1 : Inport
  " InputMux " : Subsystem
      mask Display: disp('Mux')
  " S-Function " : S-Function  FunctionName=plecs  SFunctionDeploymentMode=off  EnableBusSupport=off
  wires:
  1/1 -> " InputMux "/1(In1)
  " InputMux "/1(Out) -> " S-Function "/1

== system FOC_PMSM_FVSensorNew/PMSM motor/abc 2 dq ==
  abc : Inport
  theta : Inport  Port=2
  Mux1 : Mux  Inputs=2
  Mux2 : Mux  Inputs=2
  abc2d : Fcn  Expr=-1*2/3*(u(1)*sin(u(4))+u(2)*sin(u(4)-2*pi/3)+u(3)*sin(u(4)-4*pi/3))
  abc2q : Fcn  Expr=2/3*(u(1)*cos(u(4))+u(2)*cos(u(4)-2*pi/3)+u(3)*cos(u(4)-4*pi/3))
  dq : Outport  VectorParamsAs1DForOutWhenUnconnected=off
  wires:
  Mux2/1 -> dq/1
  abc2d/1 -> Mux2/2
  abc2q/1 -> Mux2/1
  Mux1/1 -> abc2d/1, abc2q/1
  theta/1 -> Mux1/2
  abc/1 -> Mux1/1

== system FOC_PMSM_FVSensorNew/PMSM motor/dq 2 afa beta ==
  dq : Inport
  theta : Inport  Port=2
  Mux1 : Mux  Inputs=2
  Mux2 : Mux  Inputs=2
  dq2afa : Fcn  Expr=u(1)*cos(u(3))-u(2)*sin(u(3))
  dq2beta : Fcn  Expr=u(1)*sin(u(3))+u(2)*cos(u(3))
  afa beta : Outport  VectorParamsAs1DForOutWhenUnconnected=off
  wires:
  dq/1 -> Mux1/1
  theta/1 -> Mux1/2
  Mux1/1 -> dq2beta/1, dq2afa/1
  dq2afa/1 -> Mux2/1
  dq2beta/1 -> Mux2/2
  Mux2/1 -> afa beta/1

== system FOC_PMSM_FVSensorNew/PMSM motor/dq0 2 abc ==
  dq0 : Inport
  theta : Inport  Port=2
  Mux1 : Mux  Inputs=2
  Mux2 : Mux  Inputs=3
  qd2a : Fcn  Expr=u(1)*cos(u(4))-u(2)*sin(u(4))+u(3)
  qd2b : Fcn  Expr=u(1)*cos(u(4)-2/3*pi)-u(2)*sin(u(4)-2/3*pi)+u(3)
  qd2c : Fcn  Expr=u(1)*cos(u(4)+2/3*pi)-u(2)*sin(u(4)+2/3*pi)+u(3)
  abc : Outport  VectorParamsAs1DForOutWhenUnconnected=off
  wires:
  Mux2/1 -> abc/1
  qd2b/1 -> Mux2/2
  qd2a/1 -> Mux2/1
  Mux1/1 -> qd2b/1, qd2c/1, qd2a/1
  theta/1 -> Mux1/2
  dq0/1 -> Mux1/1
  qd2c/1 -> Mux2/3

== system FOC_PMSM_FVSensorNew/PMSM motor/dq0 2 abc1 ==
  dq0 : Inport
  theta : Inport  Port=2
  Mux1 : Mux  Inputs=2
  Mux2 : Mux  Inputs=3
  qd2a : Fcn  Expr=u(1)*cos(u(4))-u(2)*sin(u(4))+u(3)
  qd2b : Fcn  Expr=u(1)*cos(u(4)-2/3*pi)-u(2)*sin(u(4)-2/3*pi)+u(3)
  qd2c : Fcn  Expr=u(1)*cos(u(4)+2/3*pi)-u(2)*sin(u(4)+2/3*pi)+u(3)
  abc : Outport  VectorParamsAs1DForOutWhenUnconnected=off
  wires:
  qd2c/1 -> Mux2/3
  dq0/1 -> Mux1/1
  theta/1 -> Mux1/2
  Mux1/1 -> qd2a/1, qd2c/1, qd2b/1
  qd2a/1 -> Mux2/1
  qd2b/1 -> Mux2/2
  Mux2/1 -> abc/1

== system FOC_PMSM_FVSensorNew/Position and speed estimation/Triggered Subsystem ==
  In1 : Inport
  theta : Inport  Port=2  LatchByDelayingOutsideSignal=on
  Trigger : TriggerPort  VariantControl=Variant
  Memory : Memory  InheritSampleTime=on
  abc 2 dq : Subsystem
  i_dq : Outport
  i_dq_old : Outport  Port=2
  wires:
  In1/1 -> abc 2 dq/1(abc)
  abc 2 dq/1(dq) -> Memory/1, i_dq/1
  Memory/1 -> i_dq_old/1
  theta/1 -> abc 2 dq/2(theta)

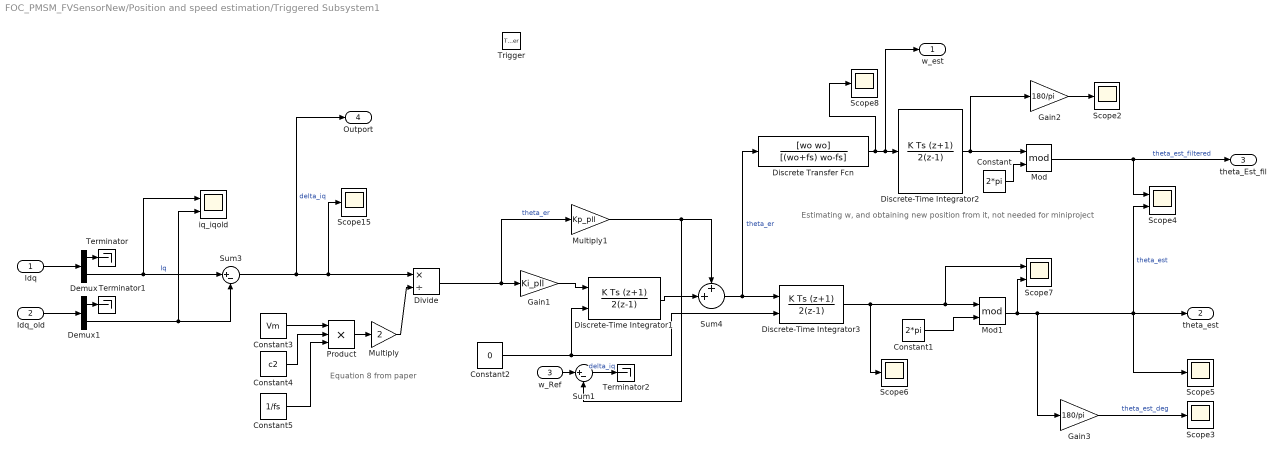
== system FOC_PMSM_FVSensorNew/Position and speed estimation/Triggered Subsystem1 ==
  note: Estimating w, and obtaining new position from it, not needed for miniproject
  note: Equation 8 from paper
  Idq : Inport
  Idq_old : Inport  Port=2
  w_Ref : Inport  Port=3
  Trigger : TriggerPort  VariantControl=Variant
  Constant : Constant  Value=2*pi
  Constant1 : Constant  Value=2*pi
  Constant2 : Constant  Value=0
  Constant3 : Constant  Value=Vm
  Constant4 : Constant  Value=c2
  Constant5 : Constant  Value=1/fs
  Demux : Demux  Outputs=2
  Demux1 : Demux  Outputs=2
  Discrete Transfer Fcn : DiscreteTransferFcn  Numerator=[wo wo]  Denominator=[(wo+fs) wo-fs]
  Discrete-Time Integrator1 : DiscreteIntegrator  IntegratorMethod=Integration: Trapezoidal  gainval=1  InitialConditionSource=external  SampleTime=-1  ICPrevOutput=DiscIntNeverNeededParam  ICPrevScaledInput=DiscIntNeverNeededParam
  Discrete-Time Integrator2 : DiscreteIntegrator  IntegratorMethod=Integration: Trapezoidal  gainval=1  SampleTime=-1  ICPrevOutput=DiscIntNeverNeededParam  ICPrevScaledInput=DiscIntNeverNeededParam
  Discrete-Time Integrator3 : DiscreteIntegrator  IntegratorMethod=Integration: Trapezoidal  gainval=1  InitialConditionSource=external  SampleTime=-1  ICPrevOutput=DiscIntNeverNeededParam  ICPrevScaledInput=DiscIntNeverNeededParam
  Divide : Product  Inputs=*/
  Gain1 : Gain  Gain=Ki_pll
  Gain2 : Gain  Gain=180/pi
  Gain3 : Gain  Gain=180/pi
  Mod : Math  Operator=mod  SignedPower=off  SaturateOnIntegerOverflow=on
  Mod1 : Math  Operator=mod  SignedPower=off  SaturateOnIntegerOverflow=on
  Multiply : Gain  Gain=2
  Multiply1 : Gain  Gain=Kp_pll
  Product : Product  Inputs=3
  Scope{2..3,5..6,8,15} (6 alike) : Scope
  Scope4 : Scope  NumInputPorts=2
  Scope7 : Scope  NumInputPorts=2
  Sum1 : Sum  Inputs=|+-
  Sum3 : Sum  Inputs=|+-
  Sum4 : Sum  Inputs=++|
  Terminator : Terminator
  Terminator1 : Terminator
  Terminator2 : Terminator
  iq_iqold : Scope  NumInputPorts=2
  w_est : Outport
  theta_est : Outport  Port=2
  theta_Est_fil : Outport  Port=3
  Outport : Outport  Port=4
  wires:
  Discrete-Time Integrator2/1 -> Mod/1, Gain2/1
  Multiply/1 -> Divide/2
  Constant4/1 -> Product/2
  Constant5/1 -> Product/3
  Product/1 -> Multiply/1
  Gain1/1 -> Discrete-Time Integrator1/1
  Constant3/1 -> Product/1
  Gain2/1 -> Scope2/1
  Constant/1 -> Mod/2
  Discrete Transfer Fcn/1 -> Scope8/1, w_est/1, Discrete-Time Integrator2/1
  Mod/1 -> theta_Est_fil/1, Scope4/1  "theta_est_filtered"
  Mod1/1 -> Scope7/2, Gain3/1, theta_est/1, Scope5/1, Scope4/2  "theta_est"
  Discrete-Time Integrator1/1 -> Sum4/2
  Constant1/1 -> Mod1/2
  Multiply1/1 -> Sum1/2, Sum4/1
  Sum3/1 -> Outport/1, Scope15/1, Divide/1  "delta_iq"
  Demux/2 -> iq_iqold/1, Sum3/1  "Iq"
  Demux1/2 -> iq_iqold/2, Sum3/2
  Discrete-Time Integrator3/1 -> Scope6/1, Scope7/1, Mod1/1
  Demux1/1 -> Terminator1/1
  Demux/1 -> Terminator/1
  Gain3/1 -> Scope3/1  "theta_est_deg"
  Idq_old/1 -> Demux1/1
  Idq/1 -> Demux/1
  w_Ref/1 -> Sum1/1
  Divide/1 -> Multiply1/1, Gain1/1  "theta_er"
  Constant2/1 -> Discrete-Time Integrator1/2, Discrete-Time Integrator3/2
  Sum1/1 -> Terminator2/1  "delta_iq"
  Sum4/1 -> Discrete Transfer Fcn/1, Discrete-Time Integrator3/1  "theta_er"

== system FOC_PMSM_FVSensorNew/Position and speed estimation/Triggered Subsystem2 ==
  In1 : Inport
  theta : Inport  Port=2  LatchByDelayingOutsideSignal=on
  Trigger : TriggerPort  VariantControl=Variant
  Memory : Memory  InheritSampleTime=on
  abc 2 dq : Subsystem
  i_dq : Outport
  i_dq_old : Outport  Port=2
  wires:
  In1/1 -> abc 2 dq/1(abc)
  abc 2 dq/1(dq) -> Memory/1, i_dq/1
  Memory/1 -> i_dq_old/1
  theta/1 -> abc 2 dq/2(theta)

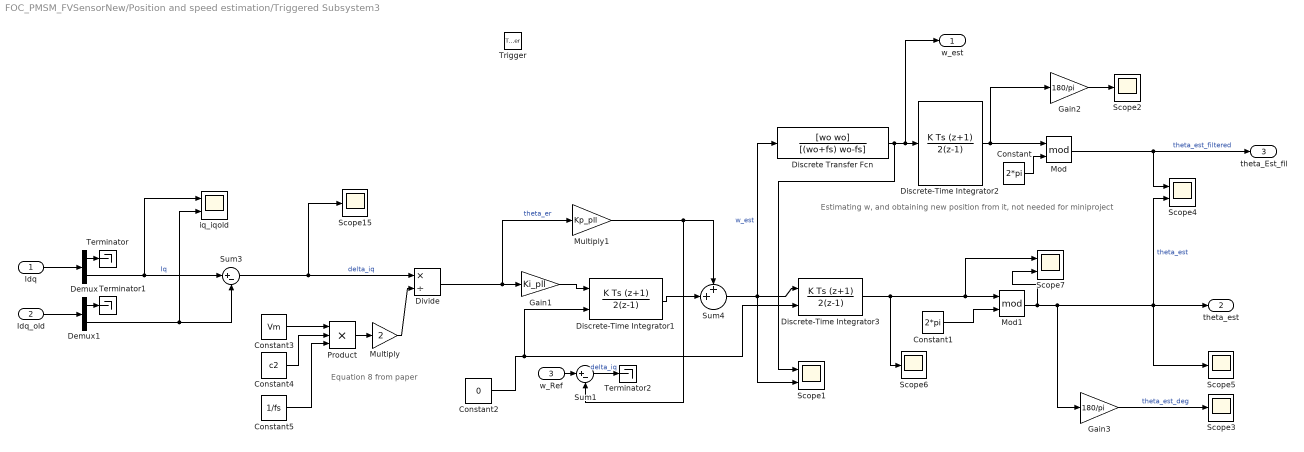
== system FOC_PMSM_FVSensorNew/Position and speed estimation/Triggered Subsystem3 ==
  note: Estimating w, and obtaining new position from it, not needed for miniproject
  note: Equation 8 from paper
  Idq : Inport
  Idq_old : Inport  Port=2
  w_Ref : Inport  Port=3
  Trigger : TriggerPort  VariantControl=Variant
  Constant : Constant  Value=2*pi
  Constant1 : Constant  Value=2*pi
  Constant2 : Constant  Value=0
  Constant3 : Constant  Value=Vm
  Constant4 : Constant  Value=c2
  Constant5 : Constant  Value=1/fs
  Demux : Demux  Outputs=2
  Demux1 : Demux  Outputs=2
  Discrete Transfer Fcn : DiscreteTransferFcn  Numerator=[wo wo]  Denominator=[(wo+fs) wo-fs]
  Discrete-Time Integrator1 : DiscreteIntegrator  IntegratorMethod=Integration: Trapezoidal  gainval=1  InitialConditionSource=external  SampleTime=-1  ICPrevOutput=DiscIntNeverNeededParam  ICPrevScaledInput=DiscIntNeverNeededParam
  Discrete-Time Integrator2 : DiscreteIntegrator  IntegratorMethod=Integration: Trapezoidal  gainval=1  SampleTime=-1  ICPrevOutput=DiscIntNeverNeededParam  ICPrevScaledInput=DiscIntNeverNeededParam
  Discrete-Time Integrator3 : DiscreteIntegrator  IntegratorMethod=Integration: Trapezoidal  gainval=1  InitialConditionSource=external  SampleTime=-1  ICPrevOutput=DiscIntNeverNeededParam  ICPrevScaledInput=DiscIntNeverNeededParam
  Divide : Product  Inputs=*/
  Gain1 : Gain  Gain=Ki_pll
  Gain2 : Gain  Gain=180/pi
  Gain3 : Gain  Gain=180/pi
  Mod : Math  Operator=mod  SignedPower=off  SaturateOnIntegerOverflow=on
  Mod1 : Math  Operator=mod  SignedPower=off  SaturateOnIntegerOverflow=on
  Multiply : Gain  Gain=2
  Multiply1 : Gain  Gain=Kp_pll
  Product : Product  Inputs=3
  Scope1 : Scope  NumInputPorts=2
  Scope{2..3,5..6,15} (5 alike) : Scope
  Scope4 : Scope  NumInputPorts=2
  Scope7 : Scope  NumInputPorts=2
  Sum1 : Sum  Inputs=|+-
  Sum3 : Sum  Inputs=|+-
  Sum4 : Sum  Inputs=++|
  Terminator : Terminator
  Terminator1 : Terminator
  Terminator2 : Terminator
  iq_iqold : Scope  NumInputPorts=2
  w_est : Outport
  theta_est : Outport  Port=2
  theta_Est_fil : Outport  Port=3
  wires:
  Discrete-Time Integrator2/1 -> Mod/1, Gain2/1
  Multiply/1 -> Divide/2
  Constant4/1 -> Product/2
  Constant5/1 -> Product/3
  Product/1 -> Multiply/1
  Gain1/1 -> Discrete-Time Integrator1/1
  Constant3/1 -> Product/1
  Gain2/1 -> Scope2/1
  Constant/1 -> Mod/2
  Discrete Transfer Fcn/1 -> Scope1/1, w_est/1, Discrete-Time Integrator2/1
  Mod/1 -> theta_Est_fil/1, Scope4/1  "theta_est_filtered"
  Mod1/1 -> Scope7/2, Gain3/1, theta_est/1, Scope5/1, Scope4/2  "theta_est"
  Discrete-Time Integrator1/1 -> Sum4/2
  Constant1/1 -> Mod1/2
  Sum4/1 -> Scope1/2, Discrete Transfer Fcn/1, Discrete-Time Integrator3/1  "w_est"
  Multiply1/1 -> Sum1/2, Sum4/1
  Sum3/1 -> Scope15/1, Divide/1  "delta_iq"
  Demux/2 -> iq_iqold/1, Sum3/1  "Iq"
  Demux1/2 -> iq_iqold/2, Sum3/2
  Discrete-Time Integrator3/1 -> Scope6/1, Scope7/1, Mod1/1
  Demux1/1 -> Terminator1/1
  Demux/1 -> Terminator/1
  Gain3/1 -> Scope3/1  "theta_est_deg"
  Idq_old/1 -> Demux1/1
  Idq/1 -> Demux/1
  w_Ref/1 -> Sum1/1
  Divide/1 -> Multiply1/1, Gain1/1  "theta_er"
  Constant2/1 -> Discrete-Time Integrator1/2, Discrete-Time Integrator3/2
  Sum1/1 -> Terminator2/1  "delta_iq"

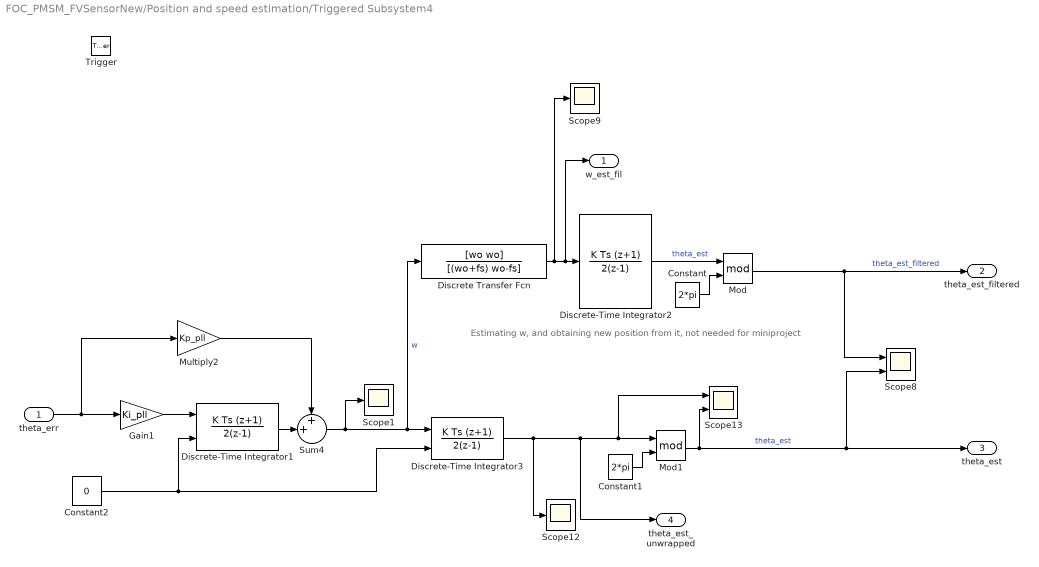
== system FOC_PMSM_FVSensorNew/Position and speed estimation/Triggered Subsystem4 ==
  note: Estimating w, and obtaining new position from it, not needed for miniproject
  theta_err : Inport
  Trigger : TriggerPort  VariantControl=Variant
  Constant : Constant  Value=2*pi
  Constant1 : Constant  Value=2*pi
  Constant2 : Constant  Value=0
  Discrete Transfer Fcn : DiscreteTransferFcn  Numerator=[wo wo]  Denominator=[(wo+fs) wo-fs]
  Discrete-Time Integrator1 : DiscreteIntegrator  IntegratorMethod=Integration: Trapezoidal  gainval=1  InitialConditionSource=external  SampleTime=-1  ICPrevOutput=DiscIntNeverNeededParam  ICPrevScaledInput=DiscIntNeverNeededParam
  Discrete-Time Integrator2 : DiscreteIntegrator  IntegratorMethod=Integration: Trapezoidal  gainval=1  SampleTime=-1  ICPrevOutput=DiscIntNeverNeededParam  ICPrevScaledInput=DiscIntNeverNeededParam
  Discrete-Time Integrator3 : DiscreteIntegrator  IntegratorMethod=Integration: Trapezoidal  gainval=1  InitialConditionSource=external  SampleTime=-1  ICPrevOutput=DiscIntNeverNeededParam  ICPrevScaledInput=DiscIntNeverNeededParam
  Gain1 : Gain  Gain=Ki_pll
  Mod : Math  Operator=mod  SignedPower=off  SaturateOnIntegerOverflow=on
  Mod1 : Math  Operator=mod  SignedPower=off  SaturateOnIntegerOverflow=on
  Multiply2 : Gain  Gain=Kp_pll
  Scope1 : Scope
  Scope12 : Scope
  Scope13 : Scope  NumInputPorts=2
  Scope8 : Scope  NumInputPorts=2
  Scope9 : Scope
  Sum4 : Sum  Inputs=++|
  w_est_fil : Outport
  theta_est_filtered : Outport  Port=2
  theta_est : Outport  Port=3
  theta_est_unwrapped : Outport  Port=4
  wires:
  Gain1/1 -> Discrete-Time Integrator1/1
  Multiply2/1 -> Sum4/1
  Mod/1 -> theta_est_filtered/1, Scope8/1  "theta_est_filtered"
  Sum4/1 -> Discrete Transfer Fcn/1, Discrete-Time Integrator3/1, Scope1/1  "w"
  Mod1/1 -> Scope13/2, Scope8/2, theta_est/1  "theta_est"
  Constant2/1 -> Discrete-Time Integrator3/2, Discrete-Time Integrator1/2
  Constant/1 -> Mod/2
  Discrete-Time Integrator3/1 -> Scope12/1, theta_est_unwrapped/1, Scope13/1, Mod1/1
  Discrete-Time Integrator1/1 -> Sum4/2
  Discrete Transfer Fcn/1 -> Scope9/1, w_est_fil/1, Discrete-Time Integrator2/1
  Constant1/1 -> Mod1/2
  Discrete-Time Integrator2/1 -> Mod/1  "theta_est"
  theta_err/1 -> Multiply2/1, Gain1/1

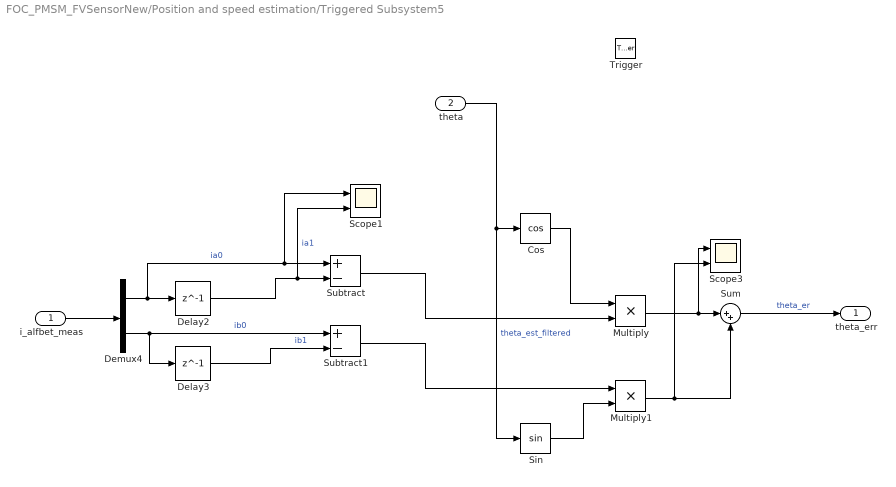
== system FOC_PMSM_FVSensorNew/Position and speed estimation/Triggered Subsystem5 ==
  i_alfbet_meas : Inport
  theta : Inport  Port=2  LatchByDelayingOutsideSignal=on
  Trigger : TriggerPort  VariantControl=Variant
  Cos : Trigonometry  Operator=cos
  Delay2 : Delay  DelayLength=1
  Delay3 : Delay  DelayLength=1
  Demux4 : Demux  Outputs=2
  Multiply : Product
  Multiply1 : Product
  Scope1 : Scope  NumInputPorts=2
  Scope3 : Scope  NumInputPorts=2
  Sin : Trigonometry
  Subtract : Sum  Inputs=+-
  Subtract1 : Sum  Inputs=+-
  Sum : Sum  Inputs=|++
  theta_err : Outport
  wires:
  Cos/1 -> Multiply/1
  Sum/1 -> theta_err/1  "theta_er"
  Sin/1 -> Multiply1/2
  Demux4/1 -> Scope1/1, Subtract/1, Delay2/1  "ia0"
  Multiply1/1 -> Sum/2, Scope3/2
  Delay3/1 -> Subtract1/2  "ib1"
  Demux4/2 -> Delay3/1, Subtract1/1  "ib0"
  i_alfbet_meas/1 -> Demux4/1
  Subtract/1 -> Multiply/2
  theta/1 -> Sin/1, Cos/1  "theta_est_filtered"
  Subtract1/1 -> Multiply1/1
  Multiply/1 -> Scope3/1, Sum/1
  Delay2/1 -> Scope1/2, Subtract/2  "ia1"

== system FOC_PMSM_FVSensorNew/Pulse injection/afabet 2 abc ==
  afabet : Inport
  Constant : Constant  Value=0
  Mux1 : Mux  Inputs=2
  Mux2 : Mux  Inputs=3
  qd2a : Fcn  Expr=u(1)+u(3)
  qd2b : Fcn  Expr=u(1)*cos(2/3*pi)+u(2)*sin(2/3*pi)+u(3)
  qd2c : Fcn  Expr=u(1)*cos(2/3*pi)-u(2)*sin(2/3*pi)+u(3)
  abc : Outport  VectorParamsAs1DForOutWhenUnconnected=off
  wires:
  Constant/1 -> Mux1/2
  qd2c/1 -> Mux2/3
  afabet/1 -> Mux1/1
  Mux1/1 -> qd2c/1, qd2b/1, qd2a/1
  qd2a/1 -> Mux2/1
  qd2b/1 -> Mux2/2
  Mux2/1 -> abc/1

== system FOC_PMSM_FVSensorNew/Pulse injection/dq 2 afa beta ==
  dq : Inport
  theta : Inport  Port=2
  Mux1 : Mux  Inputs=2
  Mux2 : Mux  Inputs=2
  dq2afa : Fcn  Expr=u(1)*cos(u(3))-u(2)*sin(u(3))
  dq2beta : Fcn  Expr=u(1)*sin(u(3))+u(2)*cos(u(3))
  afa beta : Outport  VectorParamsAs1DForOutWhenUnconnected=off
  wires:
  dq/1 -> Mux1/1
  theta/1 -> Mux1/2
  Mux1/1 -> dq2beta/1, dq2afa/1
  dq2afa/1 -> Mux2/1
  dq2beta/1 -> Mux2/2
  Mux2/1 -> afa beta/1

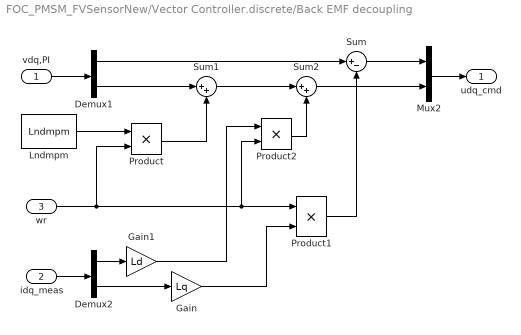
== system FOC_PMSM_FVSensorNew/Vector Controller.discrete/Back EMF decoupling ==
  vdq,PI : Inport
  idq_meas : Inport  Port=2
  wr : Inport  Port=3
  Demux1 : Demux  Outputs=2
  Demux2 : Demux  Outputs=2
  Gain : Gain  Gain=Lq
  Gain1 : Gain  Gain=Ld
  Lndmpm : Constant  Value=Lndmpm
  Mux2 : Mux  Inputs=2
  Product : Product  RndMeth=Zero
  Product1 : Product  RndMeth=Zero
  Product2 : Product  RndMeth=Zero
  Sum : Sum  Inputs=|+-
  Sum1 : Sum  Inputs=|++
  Sum2 : Sum  Inputs=|++
  udq_cmd : Outport  VectorParamsAs1DForOutWhenUnconnected=off
  wires:
  Mux2/1 -> udq_cmd/1
  vdq,PI/1 -> Demux1/1
  Demux1/1 -> Sum/1
  Sum/1 -> Mux2/1
  Demux1/2 -> Sum1/1
  idq_meas/1 -> Demux2/1
  wr/1 -> Product/2, Product1/1, Product2/2
  Product1/1 -> Sum/2
  Gain/1 -> Product1/2
  Demux2/2 -> Gain/1
  Lndmpm/1 -> Product/1
  Product/1 -> Sum1/2
  Sum1/1 -> Sum2/1
  Demux2/1 -> Gain1/1
  Gain1/1 -> Product2/1
  Product2/1 -> Sum2/2
  Sum2/1 -> Mux2/2

== system FOC_PMSM_FVSensorNew/Vector Controller.discrete/PI controller.2 ==
  id_err : Inport
  Discrete-Time Integrator : DiscreteIntegrator  SampleTime=-1  ICPrevOutput=DiscIntNeverNeededParam  ICPrevScaledInput=DiscIntNeverNeededParam
  Kp : Gain  Gain=Kp2
  Sum1 : Sum  Inputs=|++
  ki : Gain  Gain=Ki2
  vd : Outport  VectorParamsAs1DForOutWhenUnconnected=off
  wires:
  Sum1/1 -> vd/1
  Discrete-Time Integrator/1 -> Sum1/2
  ki/1 -> Discrete-Time Integrator/1
  Kp/1 -> Sum1/1
  id_err/1 -> ki/1, Kp/1

== system FOC_PMSM_FVSensorNew/Vector Controller.discrete/PI controller.3 ==
  iq_err : Inport
  Discrete-Time Integrator : DiscreteIntegrator  SampleTime=-1  ICPrevOutput=DiscIntNeverNeededParam  ICPrevScaledInput=DiscIntNeverNeededParam
  Kp : Gain  Gain=8
  Sum1 : Sum  Inputs=|++
  ki : Gain  Gain=5000
  vq : Outport  VectorParamsAs1DForOutWhenUnconnected=off
  wires:
  Sum1/1 -> vq/1
  Discrete-Time Integrator/1 -> Sum1/2
  ki/1 -> Discrete-Time Integrator/1
  Kp/1 -> Sum1/1
  iq_err/1 -> ki/1, Kp/1

== system FOC_PMSM_FVSensorNew/Vector Controller.discrete/dq 2 afa beta ==
  dq : Inport
  theta : Inport  Port=2
  Mux1 : Mux  Inputs=2
  Mux2 : Mux  Inputs=2
  dq2afa : Fcn  Expr=u(1)*cos(u(3))-u(2)*sin(u(3))
  dq2beta : Fcn  Expr=u(1)*sin(u(3))+u(2)*cos(u(3))
  afa beta : Outport  VectorParamsAs1DForOutWhenUnconnected=off
  wires:
  Mux2/1 -> afa beta/1
  dq2beta/1 -> Mux2/2
  dq2afa/1 -> Mux2/1
  Mux1/1 -> dq2afa/1, dq2beta/1
  theta/1 -> Mux1/2
  dq/1 -> Mux1/1

== system FOC_PMSM_FVSensorNew/PLL/Scope/ InputMux  ==
  In1 : Inport
  Convert1 : DataTypeConversion  SaturateOnIntegerOverflow=on  RndMeth=Zero
  Mux : Mux  Inputs=1
  Out : Outport  VectorParamsAs1DForOutWhenUnconnected=off
  wires:
  Convert1/1 -> Mux/1
  In1/1 -> Convert1/1
  Mux/1 -> Out/1

== system FOC_PMSM_FVSensorNew/PMSM motor/Scope2/ InputMux  ==
  In1 : Inport
  Convert1 : DataTypeConversion  SaturateOnIntegerOverflow=on  RndMeth=Zero
  Mux : Mux  Inputs=1
  Out : Outport  VectorParamsAs1DForOutWhenUnconnected=off
  wires:
  Convert1/1 -> Mux/1
  In1/1 -> Convert1/1
  Mux/1 -> Out/1

== system FOC_PMSM_FVSensorNew/PMSM motor/Scope3/ InputMux  ==
  In1 : Inport
  Convert1 : DataTypeConversion  SaturateOnIntegerOverflow=on  RndMeth=Zero
  Mux : Mux  Inputs=1
  Out : Outport  VectorParamsAs1DForOutWhenUnconnected=off
  wires:
  Mux/1 -> Out/1
  In1/1 -> Convert1/1
  Convert1/1 -> Mux/1

== system FOC_PMSM_FVSensorNew/PMSM motor/Scope4/ InputMux  ==
  In1 : Inport
  Convert1 : DataTypeConversion  SaturateOnIntegerOverflow=on  RndMeth=Zero
  Mux : Mux  Inputs=1
  Out : Outport  VectorParamsAs1DForOutWhenUnconnected=off
  wires:
  Convert1/1 -> Mux/1
  In1/1 -> Convert1/1
  Mux/1 -> Out/1
